simulink library "l1_blocks"  (R2026a)
settings: Solver=VariableStepAuto
PreLoadFcn:
  | run('l1_init')
undefined symbols (not defined in the file or in its folder): a_max, ctrl_den, ctrl_num, delay_samples_gps, DiscIntNeverNeededParam, dt_sim, r0, sigma_pos, sigma_vel, traj_circle_center, traj_circle_R, traj_line_dir, traj_line_origin, traj_sin_Amp, traj_sin_dir, traj_sin_freq, traj_sin_origin, V, v0, wind_vector
libraries: simulink x2
settings Model: Creator=eduno  LastModifiedBy=eduno

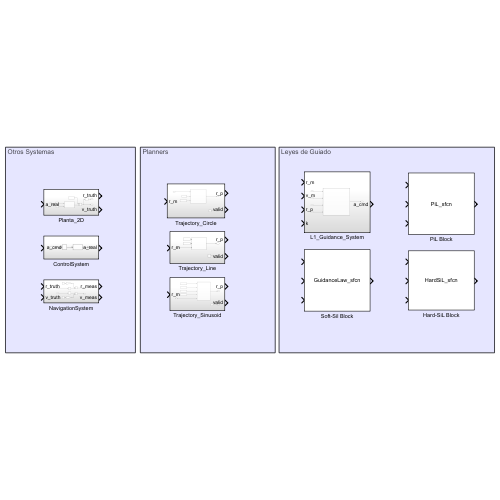
[thumbnail: Simulink's stored preview of the top-level diagram]
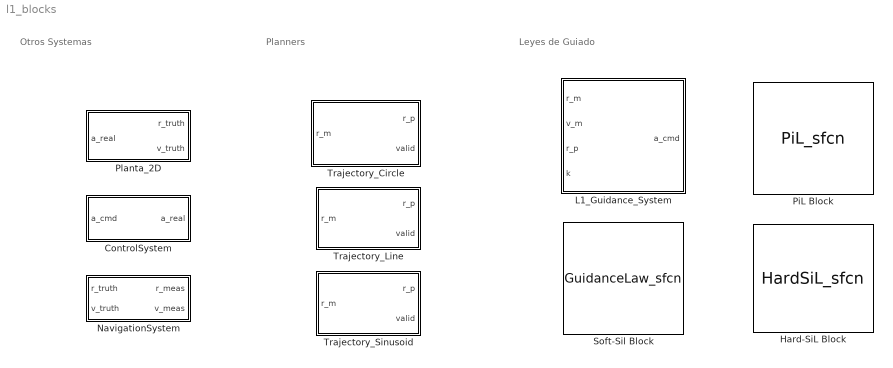
== system l1_blocks ==
  note: Otros Systemas
  note: Leyes de Guiado
  note: Planners
  ControlSystem : Subsystem
  Hard-SiL Block : S-Function  FunctionName=HardSiL_sfcn  SFunctionDeploymentMode=off  EnableBusSupport=off
  L1_Guidance_System : Subsystem
  NavigationSystem : Subsystem
  PiL Block : S-Function  FunctionName=PiL_sfcn  SFunctionDeploymentMode=off  EnableBusSupport=off
  Planta_2D : Subsystem
  Soft-Sil Block : S-Function  FunctionName=GuidanceLaw_sfcn  SFunctionDeploymentMode=off  EnableBusSupport=off
  Trajectory_Circle : Subsystem
  Trajectory_Line : Subsystem
  Trajectory_Sinusoid : Subsystem

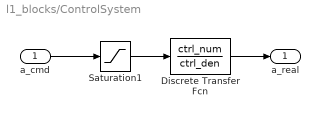
== system l1_blocks/ControlSystem ==
  " a_cmd" : Inport  PortDimensions=2
  Discrete Transfer Fcn : DiscreteTransferFcn  Numerator=ctrl_num  Denominator=ctrl_den
  Saturation1 : Saturate  UpperLimit=a_max  LowerLimit=-a_max
  a_real : Outport  PortDimensions=2
  wires:
  " a_cmd"/1 -> Saturation1/1
  Saturation1/1 -> Discrete Transfer Fcn/1
  Discrete Transfer Fcn/1 -> a_real/1

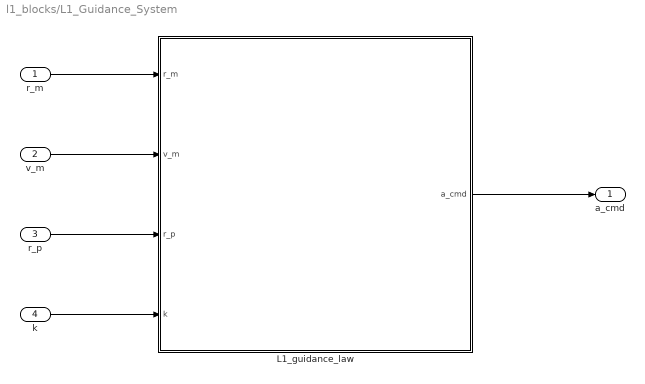
== system l1_blocks/L1_Guidance_System ==
  r_m : Inport  PortDimensions=2
  v_m : Inport  Port=2  PortDimensions=2
  r_p : Inport  Port=3  PortDimensions=2
  k : Inport  Port=4  PortDimensions=1
  L1_guidance_law : MATLAB Function  TreatAsAtomicUnit=on
  a_cmd : Outport  PortDimensions=2
  wires:
  L1_guidance_law/1(a_cmd) -> a_cmd/1
  r_p/1 -> L1_guidance_law/3(r_p)
  v_m/1 -> L1_guidance_law/2(v_m)
  r_m/1 -> L1_guidance_law/1(r_m)
  k/1 -> L1_guidance_law/4(k)

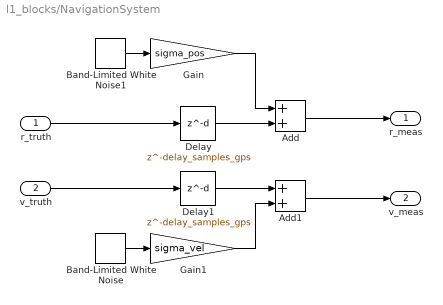
== system l1_blocks/NavigationSystem ==
  r_truth : Inport  PortDimensions=2
  v_truth : Inport  Port=2  PortDimensions=2
  Add : Sum
  Add1 : Sum
  Band-Limited White Noise : simulink/Sources/Band-Limited White Noise  Cov=[1; 1]  Ts=dt_sim  seed=seed_v
  Band-Limited White Noise1 : simulink/Sources/Band-Limited White Noise  Cov=[1; 1]  Ts=dt_sim  seed=seed_r
  Delay : Delay  DelayLength=delay_samples_gps  SampleTime=dt_sim
  Delay1 : Delay  DelayLength=delay_samples_gps  SampleTime=dt_sim
  Gain : Gain  Gain=sigma_pos
  Gain1 : Gain  Gain=sigma_vel
  r_meas : Outport  PortDimensions=2
  v_meas : Outport  Port=2  PortDimensions=2
  wires:
  r_truth/1 -> Delay/1
  v_truth/1 -> Delay1/1
  Delay/1 -> Add/2
  Add/1 -> r_meas/1
  Delay1/1 -> Add1/1
  Add1/1 -> v_meas/1
  Band-Limited White Noise1/1 -> Gain/1
  Band-Limited White Noise/1 -> Gain1/1
  Gain/1 -> Add/1
  Gain1/1 -> Add1/2

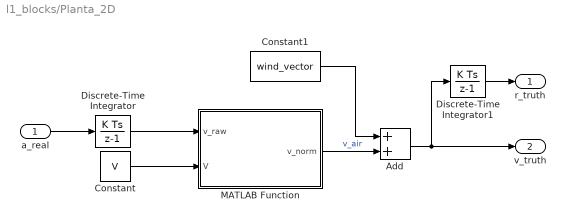
== system l1_blocks/Planta_2D ==
  a_real : Inport  PortDimensions=2
  Add : Sum
  Constant : Constant  Value=V
  Constant1 : Constant  Value=wind_vector
  Discrete-Time Integrator : DiscreteIntegrator  InitialCondition=v0  SampleTime=dt_sim  ICPrevOutput=DiscIntNeverNeededParam  ICPrevScaledInput=DiscIntNeverNeededParam
  Discrete-Time Integrator1 : DiscreteIntegrator  InitialCondition=r0  SampleTime=dt_sim  ICPrevOutput=DiscIntNeverNeededParam  ICPrevScaledInput=DiscIntNeverNeededParam
  MATLAB Function : MATLAB Function  TreatAsAtomicUnit=on
  r_truth : Outport  PortDimensions=2
  v_truth : Outport  Port=2  PortDimensions=2
  wires:
  MATLAB Function/1(v_norm) -> Add/2  "v_air"
  a_real/1 -> Discrete-Time Integrator/1
  Discrete-Time Integrator1/1 -> r_truth/1
  Discrete-Time Integrator/1 -> MATLAB Function/1(v_raw)
  Constant/1 -> MATLAB Function/2(V)
  Add/1 -> v_truth/1, Discrete-Time Integrator1/1
  Constant1/1 -> Add/1

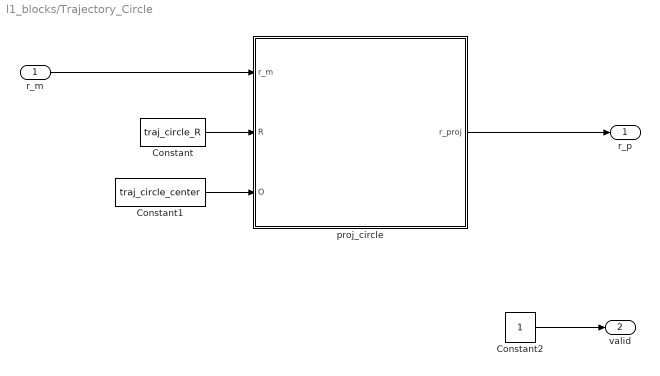
== system l1_blocks/Trajectory_Circle ==
  r_m : Inport  PortDimensions=2
  Constant : Constant  Value=traj_circle_R
  Constant1 : Constant  Value=traj_circle_center
  Constant2 : Constant
  proj_circle : MATLAB Function  TreatAsAtomicUnit=on
  r_p : Outport  PortDimensions=2
  valid : Outport  Port=2  PortDimensions=1
  wires:
  r_m/1 -> proj_circle/1(r_m)
  Constant/1 -> proj_circle/2(R)
  proj_circle/1(r_proj) -> r_p/1
  Constant1/1 -> proj_circle/3(O)
  Constant2/1 -> valid/1

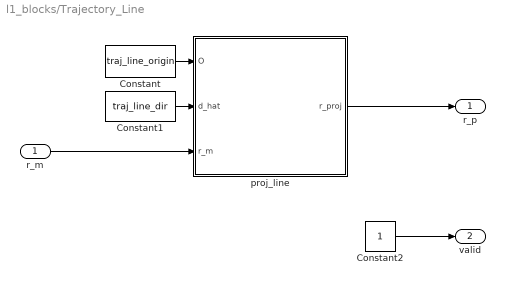
== system l1_blocks/Trajectory_Line ==
  r_m : Inport  PortDimensions=2
  Constant : Constant  Value=traj_line_origin  VectorParams1D=off
  Constant1 : Constant  Value=traj_line_dir  VectorParams1D=off
  Constant2 : Constant
  proj_line : MATLAB Function  TreatAsAtomicUnit=on
  r_p : Outport  PortDimensions=2
  valid : Outport  Port=2  PortDimensions=1
  wires:
  proj_line/1(r_proj) -> r_p/1
  r_m/1 -> proj_line/3(r_m)
  Constant/1 -> proj_line/1(O)
  Constant1/1 -> proj_line/2(d_hat)
  Constant2/1 -> valid/1

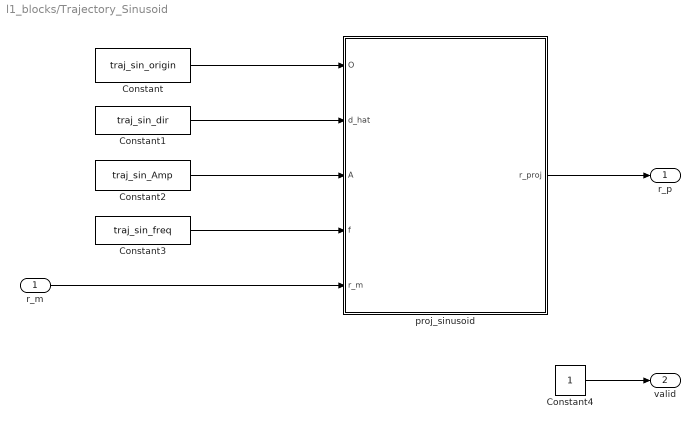
== system l1_blocks/Trajectory_Sinusoid ==
  r_m : Inport  PortDimensions=2
  Constant : Constant  Value=traj_sin_origin  VectorParams1D=off
  Constant1 : Constant  Value=traj_sin_dir
  Constant2 : Constant  Value=traj_sin_Amp
  Constant3 : Constant  Value=traj_sin_freq
  Constant4 : Constant
  proj_sinusoid : MATLAB Function  TreatAsAtomicUnit=on
  r_p : Outport  PortDimensions=2
  valid : Outport  Port=2  PortDimensions=1
  wires:
  proj_sinusoid/1(r_proj) -> r_p/1
  Constant/1 -> proj_sinusoid/1(O)
  Constant1/1 -> proj_sinusoid/2(d_hat)
  r_m/1 -> proj_sinusoid/5(r_m)
  Constant2/1 -> proj_sinusoid/3(A)
  Constant3/1 -> proj_sinusoid/4(f)
  Constant4/1 -> valid/1

== matlab function l1_blocks/L1_Guidance_System/L1_guidance_law ==
  data: r_m input; a_cmd output; v_m input; r_p input; k input
function a_cmd = L1_guidance_law(r_m, v_m, r_p, k)
% Ley de Guiado L1 [A New Nonlinear Guidance Logic for Trajectory Tracking]
%   OUT a_cmd: [2x1]    => Aceleración comandada lateral 
%                         (perpendicular a dirección de la velocidad del vehiculo)
%   IN  r_m: [2x1]      => Posición instantanea del vehiculo
%   IN  v_m: [2x1]      => Velocidad instantanea del vehiculo
%   IN  r_p: [2x1]     => Posición instantanea del punto de referencia
%                          sobre la trayectoria
%   IN  k: [1]          => Ganancia de la ley de guiado
%   
%   Formula de la ley de Guiado
%       a_cmd = k V^2 / L_1 sin(\mu)
%       - k: Ganancia
%       - V: Velocidad instantanea del vehiculo
%       - L_1: distancia hasta punto de referencia
%       - \mu: ángulo entre Velocidad y recta a punto de referencia


    L1_vec = r_p - r_m;
    L1_norm = norm(L1_vec); 
    if L1_norm < 1e-6
        a_cmd = [0; 0];
        return;
    end
    L1_hat = L1_vec / L1_norm;

    v_norm = norm(v_m);
    if v_norm < 1e-6
        a_cmd = [0; 0];
        return;
    end
    v_hat = v_m / v_norm;

    V_perp = L1_hat - dot(L1_hat, v_hat) * v_hat; 
    if norm(V_perp) < 1e-6
        a_cmd = [0; 0];
        return;
    end

    mu = acos(dot(L1_hat, v_hat));

    a_hat = V_perp/norm(V_perp);
    a_norm = k * ((v_norm^2)/L1_norm) * sin(mu);

    a_cmd = a_norm * a_hat;
end

== matlab function l1_blocks/Trajectory_Line/proj_line ==
  data: O input; d_hat input; r_proj output; r_m input
function r_proj  = proj_line(O, d_hat, r_m)
  s_proj = dot(r_m - O, d_hat);
  r_proj = O + s_proj * d_hat + 20*d_hat;
end

== matlab function l1_blocks/Planta_2D/MATLAB Function ==
  data: v_raw input; v_norm output; V input
function v_norm = normalize_velocity(v_raw, V)
    speed = norm(v_raw);
    if speed > 1e-6
        v_norm = v_raw / speed * V;
    else
        v_norm = [V; 0];
    end
end

== matlab function l1_blocks/Trajectory_Circle/proj_circle ==
  data: r_proj output; r_m input; R input; O input
function r_proj  = proj_circle(r_m, R, O)
    OM = r_m - O;
    theta_proj = atan2(OM(2), OM(1));
    r_proj = O + R * [cos(theta_proj + pi/10); sin(theta_proj + pi/10)];
end

== matlab function l1_blocks/Trajectory_Sinusoid/proj_sinusoid ==
  data: O input; d_hat input; A input; f input; r_proj output; r_m input
function r_proj  = proj_line(O, d_hat, A, f, r_m)
    s_proj = dot(r_m - O, d_hat) + 10;
    
    p = [-d_hat(2); d_hat(1)];
    p = p/norm(p);

    pert = A*sin(2*pi*f*s_proj);

    r_proj = O + s_proj * d_hat + pert * p;
end
